simulink model "A"  (R2013a)
settings: Solver=ode45  StartTime=0.0  StopTime=5  RelTol=1e-3
settings Model: Creator=Administrator  LastModifiedBy=Administrator

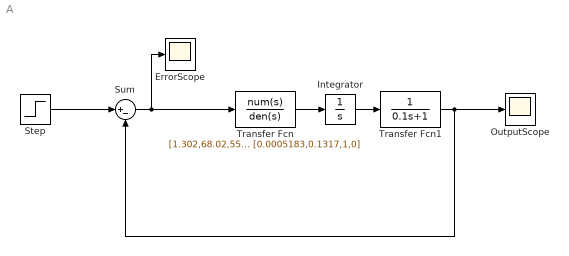
== system A ==
  ErrorScope : Scope
  Integrator : Integrator
  OutputScope : Scope
  Step : Step  SampleTime=0
  Sum : Sum  Inputs=|+-
  Transfer Fcn : TransferFcn  Numerator=[1.302,68.02,550,0]  Denominator=[0.0005183,0.1317,1,0]
  Transfer Fcn1 : TransferFcn  Denominator=[0.1 1]
  wires:
  Integrator/1 -> Transfer Fcn1/1
  Step/1 -> Sum/1
  Transfer Fcn/1 -> Integrator/1
  Transfer Fcn1/1 -> OutputScope/1, Sum/2
  Sum/1 -> Transfer Fcn/1, ErrorScope/1
